simulink model "PDPWM"  (R2013a)
settings: Solver=ode45  StartTime=0.0  StopTime=10.0  RelTol=1e-3
libraries: simulink x10
settings Model: Creator=ASUS  LastModifiedBy=ASUS

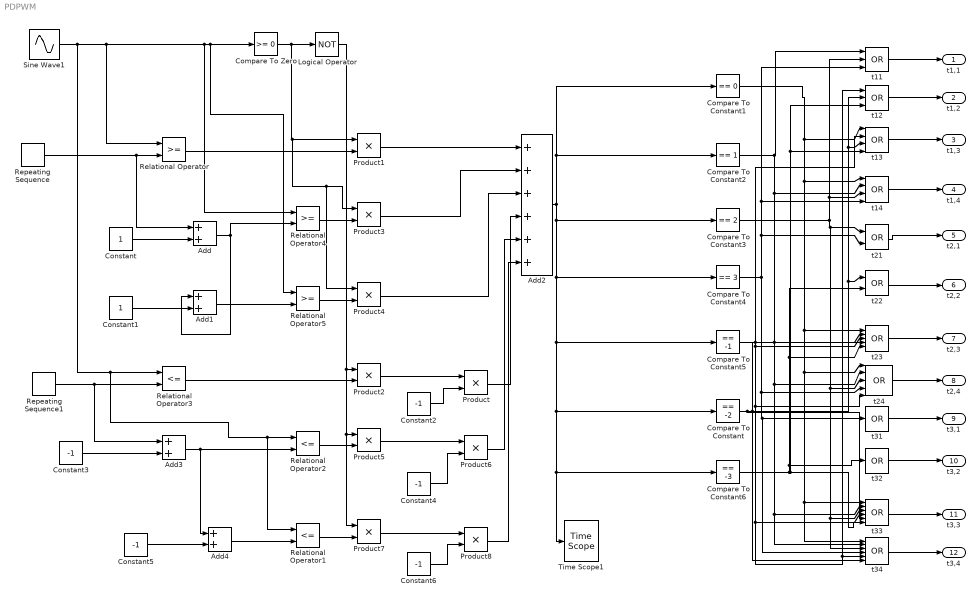
== system PDPWM ==
  Add{,1,3..4} (4 alike) : Sum
  Add2 : Sum  Inputs=++++++
  Compare To Constant : simulink/Logic and Bit Operations/Compare To Constant  relop===  const=-2  OutDataTypeStr=boolean
  Compare To Constant1 : simulink/Logic and Bit Operations/Compare To Constant  relop===  const=0  OutDataTypeStr=boolean
  Compare To Constant2 : simulink/Logic and Bit Operations/Compare To Constant  relop===  const=1  OutDataTypeStr=boolean
  Compare To Constant3 : simulink/Logic and Bit Operations/Compare To Constant  relop===  const=2  OutDataTypeStr=boolean
  Compare To Constant4 : simulink/Logic and Bit Operations/Compare To Constant  relop===  const=3  OutDataTypeStr=boolean
  Compare To Constant5 : simulink/Logic and Bit Operations/Compare To Constant  relop===  const=-1  OutDataTypeStr=boolean
  Compare To Constant6 : simulink/Logic and Bit Operations/Compare To Constant  relop===  const=-3  OutDataTypeStr=boolean
  Compare To Zero : simulink/Logic and Bit Operations/Compare To Zero  relop=>=  OutDataTypeStr=boolean
  Constant : Constant
  Constant1 : Constant
  Constant{2..6} (5 alike) : Constant  Value=-1
  Logical Operator : Logic  Operator=NOT  AllPortsSameDT=off  OutDataTypeStr=boolean
  Product{,1..8} (9 alike) : Product
  Relational Operator : RelationalOperator  OutDataTypeStr=boolean  ZeroCross=off
  Relational Operator1 : RelationalOperator  Operator=<=  OutDataTypeStr=boolean
  Relational Operator2 : RelationalOperator  Operator=<=  OutDataTypeStr=boolean
  Relational Operator3 : RelationalOperator  Operator=<=  OutDataTypeStr=boolean
  Relational Operator4 : RelationalOperator  OutDataTypeStr=boolean  ZeroCross=off
  Relational Operator5 : RelationalOperator  OutDataTypeStr=boolean  ZeroCross=off
  Repeating Sequence : simulink/Sources/Repeating Sequence  rep_seq_t=[0 1/1600 1/800]  rep_seq_y=[1 0 1]
  Repeating Sequence1 : simulink/Sources/Repeating Sequence  rep_seq_t=[0 1/1800 1/900]  rep_seq_y=[0 -1 0]
  Sine Wave1 : Sin  Amplitude=3  Frequency=2*pi*50  SampleTime=0
  Time Scope1 : TimeScope  DefaultConfigurationName=spbscopes.TimeScopeBlockCfg
      settings: CopyFcn=scopeextensions.ScopeBlock.callback(gcbh, 'onBlockCopy', gcbh);  DeleteFcn=scopeextensions.ScopeBlock.callback(gcbh, 'onBlockDelete');  PreSaveFcn=scopeextensions.ScopeBlock.callback(gcbh, 'onModelSave');  NameChangeFcn=scopeextensions.ScopeBlock.callback(gcbh, 'onBlockRename');  CloseFcn=scopeextensions.ScopeBlock.callback(gcbh, 'onBlockClose');  PreDeleteFcn=scopeextensions.ScopeBlock.callback(gcbh, 'onBlockPreDelete');
  t11 : Logic  Operator=OR  Inputs=3  AllPortsSameDT=off  OutDataTypeStr=boolean
  t12 : Logic  Operator=OR  Inputs=3  AllPortsSameDT=off  OutDataTypeStr=boolean
  t13 : Logic  Operator=OR  Inputs=4  AllPortsSameDT=off  OutDataTypeStr=boolean
  t14 : Logic  Operator=OR  Inputs=4  AllPortsSameDT=off  OutDataTypeStr=boolean
  t21 : Logic  Operator=OR  AllPortsSameDT=off  OutDataTypeStr=boolean
  t22 : Logic  Operator=OR  AllPortsSameDT=off  OutDataTypeStr=boolean
  t23 : Logic  Operator=OR  Inputs=5  AllPortsSameDT=off  OutDataTypeStr=boolean
  t24 : Logic  Operator=OR  Inputs=5  AllPortsSameDT=off  OutDataTypeStr=boolean
  t31 : Logic  Operator=OR  Inputs=1  AllPortsSameDT=off  OutDataTypeStr=boolean
  t32 : Logic  Operator=OR  Inputs=1  AllPortsSameDT=off  OutDataTypeStr=boolean
  t33 : Logic  Operator=OR  Inputs=6  AllPortsSameDT=off  OutDataTypeStr=boolean
  t34 : Logic  Operator=OR  Inputs=6  AllPortsSameDT=off  OutDataTypeStr=boolean
  t1,1 : Outport
  t1,2 : Outport  Port=2
  t1,3 : Outport  Port=3
  t1,4 : Outport  Port=4
  t2,1 : Outport  Port=5
  t2,2 : Outport  Port=6
  t2,3 : Outport  Port=7
  t2,4 : Outport  Port=8
  t3,1 : Outport  Port=9
  t3,2 : Outport  Port=10
  t3,3 : Outport  Port=11
  t3,4 : Outport  Port=12
  wires:
  Sine Wave1/1 -> Relational Operator1/1, Relational Operator2/1, Relational Operator3/1, Relational Operator/1, Relational Operator4/1, Relational Operator5/1, Compare To Zero/1
  Compare To Zero/1 -> Product4/1, Product3/1, Product1/1, Logical Operator/1
  Constant/1 -> Add/2
  Relational Operator/1 -> Product1/2
  Add/1 -> Relational Operator4/2, Add1/1
  Relational Operator4/1 -> Product3/2
  Constant1/1 -> Add1/2
  Add1/1 -> Relational Operator5/2
  Relational Operator5/1 -> Product4/2
  Product1/1 -> Add2/1
  Product3/1 -> Add2/2
  Repeating Sequence1/1 -> Add3/1, Relational Operator3/2
  Relational Operator3/1 -> Product2/2
  Logical Operator/1 -> Product7/1, Product5/1, Product2/1
  Constant2/1 -> Product/2
  Product2/1 -> Product/1
  Constant3/1 -> Add3/2
  Add3/1 -> Add4/1, Relational Operator2/2
  Relational Operator2/1 -> Product5/2
  Constant4/1 -> Product6/2
  Product5/1 -> Product6/1
  Constant5/1 -> Add4/2
  Add4/1 -> Relational Operator1/2
  Relational Operator1/1 -> Product7/2
  Product7/1 -> Product8/1
  Constant6/1 -> Product8/2
  Add2/1 -> Compare To Constant2/1, Compare To Constant1/1, Compare To Constant3/1, Compare To Constant4/1, Compare To Constant5/1, Compare To Constant6/1, Time Scope1/1, Compare To Constant/1
  Repeating Sequence/1 -> Add/1, Relational Operator/2
  Product4/1 -> Add2/3
  Product/1 -> Add2/4
  Product6/1 -> Add2/5
  Product8/1 -> Add2/6
  Compare To Constant1/1 -> t23/1, t24/1, t33/1, t34/1, t14/1, t13/1
  Compare To Constant2/1 -> t23/2, t34/2, t33/2, t24/2, t14/2, t11/1
  Compare To Constant3/1 -> t14/3, t11/2, t34/3, t33/3, t24/3, t21/1
  Compare To Constant4/1 -> t34/4, t31/1, t24/4, t21/2, t14/4, t11/3
  Compare To Constant5/1 -> t24/5, t33/4, t34/5, t12/1, t23/3, t13/2
  Compare To Constant/1 -> t34/6, t23/4, t22/1, t13/3, t12/2, t33/5
  Compare To Constant6/1 -> t33/6, t13/4, t12/3, t32/1, t23/5, t22/2
  t11/1 -> t1,1/1
  t12/1 -> t1,2/1
  t13/1 -> t1,3/1
  t14/1 -> t1,4/1
  t21/1 -> t2,1/1
  t22/1 -> t2,2/1
  t24/1 -> t2,4/1
  t23/1 -> t2,3/1
  t31/1 -> t3,1/1
  t32/1 -> t3,2/1
  t33/1 -> t3,3/1
  t34/1 -> t3,4/1
